simulink model "xblock_half_band_Model"  (Simulink 7.4)
settings: Solver=ode45  StartTime=0.0  StopTime=10.0  RelTol=1e-3
libraries: xbsIndex_r4 x629, casper_library_misc x12
(part 3 of 6)

== system xblock_half_band_Model/Subsystem/parallel_fir/f1/imag_sum ==
  sync : Inport
  din_1 : Inport  Port=2
  din_2 : Inport  Port=3
  din_3 : Inport  Port=4
  din_4 : Inport  Port=5
  din_5 : Inport  Port=6
  din_6 : Inport  Port=7
  din_7 : Inport  Port=8
  din_8 : Inport  Port=9
  din_9 : Inport  Port=10
  sync_delay : xbsIndex_r4/Delay  en=off  latency=4  dbl_ovrd=off  reg_retiming=off  block_type=delay
      settings: block_version=11.4
  zero_in : xbsIndex_r4/Constant  arith_type=Unsigned  const=0  n_bits=18  bin_pt=17  explicit_period=off  period=1  equ=P=C  opselect=C  inp2=PCIN>>17  opr=+  inp1=P  carry=CIN  dbl_ovrd=off  block_type=constant
      settings: block_version=11.4
  sync_out : Outport
  dout : Outport  Port=2
  wires:
  sync/1 -> sync_delay/1
  sync_delay/1 -> sync_out/1

== system xblock_half_band_Model/Subsystem/parallel_fir/f1/real_sum ==
  sync : Inport
  din_1 : Inport  Port=2
  din_2 : Inport  Port=3
  din_3 : Inport  Port=4
  din_4 : Inport  Port=5
  din_5 : Inport  Port=6
  din_6 : Inport  Port=7
  din_7 : Inport  Port=8
  din_8 : Inport  Port=9
  din_9 : Inport  Port=10
  sync_delay : xbsIndex_r4/Delay  en=off  latency=4  dbl_ovrd=off  reg_retiming=off  block_type=delay
      settings: block_version=11.4
  zero_in : xbsIndex_r4/Constant  arith_type=Unsigned  const=0  n_bits=18  bin_pt=17  explicit_period=off  period=1  equ=P=C  opselect=C  inp2=PCIN>>17  opr=+  inp1=P  carry=CIN  dbl_ovrd=off  block_type=constant
      settings: block_version=11.4
  sync_out : Outport
  dout : Outport  Port=2
  wires:
  sync/1 -> sync_delay/1
  sync_delay/1 -> sync_out/1

== system xblock_half_band_Model/Subsystem/parallel_fir1/f0/fir_col1 ==
  real1 : Inport
  imag1 : Inport  Port=2
  fir_tap1 : Subsystem
  real_out1 : Outport
  imag_out1 : Outport  Port=2
  real_sum : Outport  Port=3
  imag_sum : Outport  Port=4
  wires:
  fir_tap1/4(imag) -> imag_sum/1  "xlsub5_fir_tap1_image"
  fir_tap1/1(a_out) -> real_out1/1
  real1/1 -> fir_tap1/1(a)
  imag1/1 -> fir_tap1/2(b)
  fir_tap1/2(b_out) -> imag_out1/1
  fir_tap1/3(real) -> real_sum/1  "xlsub5_fir_tap1_real"

== system xblock_half_band_Model/Subsystem/parallel_fir1/f0/fir_col2 ==
  real1 : Inport
  imag1 : Inport  Port=2
  fir_tap1 : Subsystem
  real_out1 : Outport
  imag_out1 : Outport  Port=2
  real_sum : Outport  Port=3
  imag_sum : Outport  Port=4
  wires:
  fir_tap1/4(imag) -> imag_sum/1  "xlsub5_fir_tap1_image"
  fir_tap1/1(a_out) -> real_out1/1
  real1/1 -> fir_tap1/1(a)
  imag1/1 -> fir_tap1/2(b)
  fir_tap1/2(b_out) -> imag_out1/1
  fir_tap1/3(real) -> real_sum/1  "xlsub5_fir_tap1_real"

== system xblock_half_band_Model/Subsystem/parallel_fir1/f0/fir_col3 ==
  real1 : Inport
  imag1 : Inport  Port=2
  fir_tap1 : Subsystem
  real_out1 : Outport
  imag_out1 : Outport  Port=2
  real_sum : Outport  Port=3
  imag_sum : Outport  Port=4
  wires:
  fir_tap1/4(imag) -> imag_sum/1  "xlsub5_fir_tap1_image"
  fir_tap1/1(a_out) -> real_out1/1
  real1/1 -> fir_tap1/1(a)
  imag1/1 -> fir_tap1/2(b)
  fir_tap1/2(b_out) -> imag_out1/1
  fir_tap1/3(real) -> real_sum/1  "xlsub5_fir_tap1_real"

== system xblock_half_band_Model/Subsystem/parallel_fir1/f0/fir_col4 ==
  real1 : Inport
  imag1 : Inport  Port=2
  fir_tap1 : Subsystem
  real_out1 : Outport
  imag_out1 : Outport  Port=2
  real_sum : Outport  Port=3
  imag_sum : Outport  Port=4
  wires:
  fir_tap1/4(imag) -> imag_sum/1  "xlsub5_fir_tap1_image"
  fir_tap1/1(a_out) -> real_out1/1
  real1/1 -> fir_tap1/1(a)
  imag1/1 -> fir_tap1/2(b)
  fir_tap1/2(b_out) -> imag_out1/1
  fir_tap1/3(real) -> real_sum/1  "xlsub5_fir_tap1_real"

== system xblock_half_band_Model/Subsystem/parallel_fir1/f0/fir_col5 ==
  real1 : Inport
  imag1 : Inport  Port=2
  fir_tap1 : Subsystem
  real_out1 : Outport
  imag_out1 : Outport  Port=2
  real_sum : Outport  Port=3
  imag_sum : Outport  Port=4
  wires:
  fir_tap1/4(imag) -> imag_sum/1  "xlsub5_fir_tap1_image"
  fir_tap1/1(a_out) -> real_out1/1
  real1/1 -> fir_tap1/1(a)
  imag1/1 -> fir_tap1/2(b)
  fir_tap1/2(b_out) -> imag_out1/1
  fir_tap1/3(real) -> real_sum/1  "xlsub5_fir_tap1_real"

== system xblock_half_band_Model/Subsystem/parallel_fir1/f0/fir_col6 ==
  real1 : Inport
  imag1 : Inport  Port=2
  fir_tap1 : Subsystem
  real_out1 : Outport
  imag_out1 : Outport  Port=2
  real_sum : Outport  Port=3
  imag_sum : Outport  Port=4
  wires:
  fir_tap1/4(imag) -> imag_sum/1  "xlsub5_fir_tap1_image"
  fir_tap1/1(a_out) -> real_out1/1
  real1/1 -> fir_tap1/1(a)
  imag1/1 -> fir_tap1/2(b)
  fir_tap1/2(b_out) -> imag_out1/1
  fir_tap1/3(real) -> real_sum/1  "xlsub5_fir_tap1_real"

== system xblock_half_band_Model/Subsystem/parallel_fir1/f0/fir_col7 ==
  real1 : Inport
  imag1 : Inport  Port=2
  fir_tap1 : Subsystem
  real_out1 : Outport
  imag_out1 : Outport  Port=2
  real_sum : Outport  Port=3
  imag_sum : Outport  Port=4
  wires:
  fir_tap1/4(imag) -> imag_sum/1  "xlsub5_fir_tap1_image"
  fir_tap1/1(a_out) -> real_out1/1
  real1/1 -> fir_tap1/1(a)
  imag1/1 -> fir_tap1/2(b)
  fir_tap1/2(b_out) -> imag_out1/1
  fir_tap1/3(real) -> real_sum/1  "xlsub5_fir_tap1_real"

== system xblock_half_band_Model/Subsystem/parallel_fir1/f0/fir_col8 ==
  real1 : Inport
  imag1 : Inport  Port=2
  fir_tap1 : Subsystem
  real_out1 : Outport
  imag_out1 : Outport  Port=2
  real_sum : Outport  Port=3
  imag_sum : Outport  Port=4
  wires:
  fir_tap1/4(imag) -> imag_sum/1  "xlsub5_fir_tap1_image"
  fir_tap1/1(a_out) -> real_out1/1
  real1/1 -> fir_tap1/1(a)
  imag1/1 -> fir_tap1/2(b)
  fir_tap1/2(b_out) -> imag_out1/1
  fir_tap1/3(real) -> real_sum/1  "xlsub5_fir_tap1_real"

== system xblock_half_band_Model/Subsystem/parallel_fir1/f0/imag_sum ==
  sync : Inport
  din_1 : Inport  Port=2
  din_2 : Inport  Port=3
  din_3 : Inport  Port=4
  din_4 : Inport  Port=5
  din_5 : Inport  Port=6
  din_6 : Inport  Port=7
  din_7 : Inport  Port=8
  din_8 : Inport  Port=9
  din_9 : Inport  Port=10
  sync_delay : xbsIndex_r4/Delay  en=off  latency=4  dbl_ovrd=off  reg_retiming=off  block_type=delay
      settings: block_version=11.4
  zero_in : xbsIndex_r4/Constant  arith_type=Unsigned  const=0  n_bits=18  bin_pt=17  explicit_period=off  period=1  equ=P=C  opselect=C  inp2=PCIN>>17  opr=+  inp1=P  carry=CIN  dbl_ovrd=off  block_type=constant
      settings: block_version=11.4
  sync_out : Outport
  dout : Outport  Port=2
  wires:
  sync/1 -> sync_delay/1
  sync_delay/1 -> sync_out/1

== system xblock_half_band_Model/Subsystem/parallel_fir1/f0/real_sum ==
  sync : Inport
  din_1 : Inport  Port=2
  din_2 : Inport  Port=3
  din_3 : Inport  Port=4
  din_4 : Inport  Port=5
  din_5 : Inport  Port=6
  din_6 : Inport  Port=7
  din_7 : Inport  Port=8
  din_8 : Inport  Port=9
  din_9 : Inport  Port=10
  sync_delay : xbsIndex_r4/Delay  en=off  latency=4  dbl_ovrd=off  reg_retiming=off  block_type=delay
      settings: block_version=11.4
  zero_in : xbsIndex_r4/Constant  arith_type=Unsigned  const=0  n_bits=18  bin_pt=17  explicit_period=off  period=1  equ=P=C  opselect=C  inp2=PCIN>>17  opr=+  inp1=P  carry=CIN  dbl_ovrd=off  block_type=constant
      settings: block_version=11.4
  sync_out : Outport
  dout : Outport  Port=2
  wires:
  sync/1 -> sync_delay/1
  sync_delay/1 -> sync_out/1

== system xblock_half_band_Model/Subsystem/parallel_fir1/f0pf1/fir_col1 ==
  real1 : Inport
  imag1 : Inport  Port=2
  fir_tap1 : Subsystem
  real_out1 : Outport
  imag_out1 : Outport  Port=2
  real_sum : Outport  Port=3
  imag_sum : Outport  Port=4
  wires:
  fir_tap1/4(imag) -> imag_sum/1  "xlsub5_fir_tap1_image"
  fir_tap1/1(a_out) -> real_out1/1
  real1/1 -> fir_tap1/1(a)
  imag1/1 -> fir_tap1/2(b)
  fir_tap1/2(b_out) -> imag_out1/1
  fir_tap1/3(real) -> real_sum/1  "xlsub5_fir_tap1_real"

== system xblock_half_band_Model/Subsystem/parallel_fir1/f0pf1/fir_col2 ==
  real1 : Inport
  imag1 : Inport  Port=2
  fir_tap1 : Subsystem
  real_out1 : Outport
  imag_out1 : Outport  Port=2
  real_sum : Outport  Port=3
  imag_sum : Outport  Port=4
  wires:
  fir_tap1/4(imag) -> imag_sum/1  "xlsub5_fir_tap1_image"
  fir_tap1/1(a_out) -> real_out1/1
  real1/1 -> fir_tap1/1(a)
  imag1/1 -> fir_tap1/2(b)
  fir_tap1/2(b_out) -> imag_out1/1
  fir_tap1/3(real) -> real_sum/1  "xlsub5_fir_tap1_real"

== system xblock_half_band_Model/Subsystem/parallel_fir1/f0pf1/fir_col3 ==
  real1 : Inport
  imag1 : Inport  Port=2
  fir_tap1 : Subsystem
  real_out1 : Outport
  imag_out1 : Outport  Port=2
  real_sum : Outport  Port=3
  imag_sum : Outport  Port=4
  wires:
  fir_tap1/4(imag) -> imag_sum/1  "xlsub5_fir_tap1_image"
  fir_tap1/1(a_out) -> real_out1/1
  real1/1 -> fir_tap1/1(a)
  imag1/1 -> fir_tap1/2(b)
  fir_tap1/2(b_out) -> imag_out1/1
  fir_tap1/3(real) -> real_sum/1  "xlsub5_fir_tap1_real"

== system xblock_half_band_Model/Subsystem/parallel_fir1/f0pf1/fir_col4 ==
  real1 : Inport
  imag1 : Inport  Port=2
  fir_tap1 : Subsystem
  real_out1 : Outport
  imag_out1 : Outport  Port=2
  real_sum : Outport  Port=3
  imag_sum : Outport  Port=4
  wires:
  fir_tap1/4(imag) -> imag_sum/1  "xlsub5_fir_tap1_image"
  fir_tap1/1(a_out) -> real_out1/1
  real1/1 -> fir_tap1/1(a)
  imag1/1 -> fir_tap1/2(b)
  fir_tap1/2(b_out) -> imag_out1/1
  fir_tap1/3(real) -> real_sum/1  "xlsub5_fir_tap1_real"

== system xblock_half_band_Model/Subsystem/parallel_fir1/f0pf1/fir_col5 ==
  real1 : Inport
  imag1 : Inport  Port=2
  fir_tap1 : Subsystem
  real_out1 : Outport
  imag_out1 : Outport  Port=2
  real_sum : Outport  Port=3
  imag_sum : Outport  Port=4
  wires:
  fir_tap1/4(imag) -> imag_sum/1  "xlsub5_fir_tap1_image"
  fir_tap1/1(a_out) -> real_out1/1
  real1/1 -> fir_tap1/1(a)
  imag1/1 -> fir_tap1/2(b)
  fir_tap1/2(b_out) -> imag_out1/1
  fir_tap1/3(real) -> real_sum/1  "xlsub5_fir_tap1_real"

== system xblock_half_band_Model/Subsystem/parallel_fir1/f0pf1/imag_sum ==
  sync : Inport
  din_1 : Inport  Port=2
  din_2 : Inport  Port=3
  din_3 : Inport  Port=4
  din_4 : Inport  Port=5
  din_5 : Inport  Port=6
  din_6 : Inport  Port=7
  sync_delay : xbsIndex_r4/Delay  en=off  latency=3  dbl_ovrd=off  reg_retiming=off  block_type=delay
      settings: block_version=11.4
  zero_in : xbsIndex_r4/Constant  arith_type=Unsigned  const=0  n_bits=18  bin_pt=17  explicit_period=off  period=1  equ=P=C  opselect=C  inp2=PCIN>>17  opr=+  inp1=P  carry=CIN  dbl_ovrd=off  block_type=constant
      settings: block_version=11.4
  sync_out : Outport
  dout : Outport  Port=2
  wires:
  sync/1 -> sync_delay/1
  sync_delay/1 -> sync_out/1

== system xblock_half_band_Model/Subsystem/parallel_fir1/f0pf1/real_sum ==
  sync : Inport
  din_1 : Inport  Port=2
  din_2 : Inport  Port=3
  din_3 : Inport  Port=4
  din_4 : Inport  Port=5
  din_5 : Inport  Port=6
  din_6 : Inport  Port=7
  sync_delay : xbsIndex_r4/Delay  en=off  latency=3  dbl_ovrd=off  reg_retiming=off  block_type=delay
      settings: block_version=11.4
  zero_in : xbsIndex_r4/Constant  arith_type=Unsigned  const=0  n_bits=18  bin_pt=17  explicit_period=off  period=1  equ=P=C  opselect=C  inp2=PCIN>>17  opr=+  inp1=P  carry=CIN  dbl_ovrd=off  block_type=constant
      settings: block_version=11.4
  sync_out : Outport
  dout : Outport  Port=2
  wires:
  sync/1 -> sync_delay/1
  sync_delay/1 -> sync_out/1

== system xblock_half_band_Model/Subsystem/parallel_fir1/f1/fir_col1 ==
  real1 : Inport
  imag1 : Inport  Port=2
  fir_tap1 : Subsystem
  real_out1 : Outport
  imag_out1 : Outport  Port=2
  real_sum : Outport  Port=3
  imag_sum : Outport  Port=4
  wires:
  fir_tap1/4(imag) -> imag_sum/1  "xlsub5_fir_tap1_image"
  fir_tap1/1(a_out) -> real_out1/1
  real1/1 -> fir_tap1/1(a)
  imag1/1 -> fir_tap1/2(b)
  fir_tap1/2(b_out) -> imag_out1/1
  fir_tap1/3(real) -> real_sum/1  "xlsub5_fir_tap1_real"

== system xblock_half_band_Model/Subsystem/parallel_fir1/f1/fir_col2 ==
  real1 : Inport
  imag1 : Inport  Port=2
  fir_tap1 : Subsystem
  real_out1 : Outport
  imag_out1 : Outport  Port=2
  real_sum : Outport  Port=3
  imag_sum : Outport  Port=4
  wires:
  fir_tap1/4(imag) -> imag_sum/1  "xlsub5_fir_tap1_image"
  fir_tap1/1(a_out) -> real_out1/1
  real1/1 -> fir_tap1/1(a)
  imag1/1 -> fir_tap1/2(b)
  fir_tap1/2(b_out) -> imag_out1/1
  fir_tap1/3(real) -> real_sum/1  "xlsub5_fir_tap1_real"

== system xblock_half_band_Model/Subsystem/parallel_fir1/f1/fir_col3 ==
  real1 : Inport
  imag1 : Inport  Port=2
  fir_tap1 : Subsystem
  real_out1 : Outport
  imag_out1 : Outport  Port=2
  real_sum : Outport  Port=3
  imag_sum : Outport  Port=4
  wires:
  fir_tap1/4(imag) -> imag_sum/1  "xlsub5_fir_tap1_image"
  fir_tap1/1(a_out) -> real_out1/1
  real1/1 -> fir_tap1/1(a)
  imag1/1 -> fir_tap1/2(b)
  fir_tap1/2(b_out) -> imag_out1/1
  fir_tap1/3(real) -> real_sum/1  "xlsub5_fir_tap1_real"

== system xblock_half_band_Model/Subsystem/parallel_fir1/f1/fir_col4 ==
  real1 : Inport
  imag1 : Inport  Port=2
  fir_tap1 : Subsystem
  real_out1 : Outport
  imag_out1 : Outport  Port=2
  real_sum : Outport  Port=3
  imag_sum : Outport  Port=4
  wires:
  fir_tap1/4(imag) -> imag_sum/1  "xlsub5_fir_tap1_image"
  fir_tap1/1(a_out) -> real_out1/1
  real1/1 -> fir_tap1/1(a)
  imag1/1 -> fir_tap1/2(b)
  fir_tap1/2(b_out) -> imag_out1/1
  fir_tap1/3(real) -> real_sum/1  "xlsub5_fir_tap1_real"

== system xblock_half_band_Model/Subsystem/parallel_fir1/f1/fir_col5 ==
  real1 : Inport
  imag1 : Inport  Port=2
  fir_tap1 : Subsystem
  real_out1 : Outport
  imag_out1 : Outport  Port=2
  real_sum : Outport  Port=3
  imag_sum : Outport  Port=4
  wires:
  fir_tap1/4(imag) -> imag_sum/1  "xlsub5_fir_tap1_image"
  fir_tap1/1(a_out) -> real_out1/1
  real1/1 -> fir_tap1/1(a)
  imag1/1 -> fir_tap1/2(b)
  fir_tap1/2(b_out) -> imag_out1/1
  fir_tap1/3(real) -> real_sum/1  "xlsub5_fir_tap1_real"

== system xblock_half_band_Model/Subsystem/parallel_fir1/f1/fir_col6 ==
  real1 : Inport
  imag1 : Inport  Port=2
  fir_tap1 : Subsystem
  real_out1 : Outport
  imag_out1 : Outport  Port=2
  real_sum : Outport  Port=3
  imag_sum : Outport  Port=4
  wires:
  fir_tap1/4(imag) -> imag_sum/1  "xlsub5_fir_tap1_image"
  fir_tap1/1(a_out) -> real_out1/1
  real1/1 -> fir_tap1/1(a)
  imag1/1 -> fir_tap1/2(b)
  fir_tap1/2(b_out) -> imag_out1/1
  fir_tap1/3(real) -> real_sum/1  "xlsub5_fir_tap1_real"

== system xblock_half_band_Model/Subsystem/parallel_fir1/f1/fir_col7 ==
  real1 : Inport
  imag1 : Inport  Port=2
  fir_tap1 : Subsystem
  real_out1 : Outport
  imag_out1 : Outport  Port=2
  real_sum : Outport  Port=3
  imag_sum : Outport  Port=4
  wires:
  fir_tap1/4(imag) -> imag_sum/1  "xlsub5_fir_tap1_image"
  fir_tap1/1(a_out) -> real_out1/1
  real1/1 -> fir_tap1/1(a)
  imag1/1 -> fir_tap1/2(b)
  fir_tap1/2(b_out) -> imag_out1/1
  fir_tap1/3(real) -> real_sum/1  "xlsub5_fir_tap1_real"

== system xblock_half_band_Model/Subsystem/parallel_fir1/f1/fir_col8 ==
  real1 : Inport
  imag1 : Inport  Port=2
  fir_tap1 : Subsystem
  real_out1 : Outport
  imag_out1 : Outport  Port=2
  real_sum : Outport  Port=3
  imag_sum : Outport  Port=4
  wires:
  fir_tap1/4(imag) -> imag_sum/1  "xlsub5_fir_tap1_image"
  fir_tap1/1(a_out) -> real_out1/1
  real1/1 -> fir_tap1/1(a)
  imag1/1 -> fir_tap1/2(b)
  fir_tap1/2(b_out) -> imag_out1/1
  fir_tap1/3(real) -> real_sum/1  "xlsub5_fir_tap1_real"

== system xblock_half_band_Model/Subsystem/parallel_fir1/f1/imag_sum ==
  sync : Inport
  din_1 : Inport  Port=2
  din_2 : Inport  Port=3
  din_3 : Inport  Port=4
  din_4 : Inport  Port=5
  din_5 : Inport  Port=6
  din_6 : Inport  Port=7
  din_7 : Inport  Port=8
  din_8 : Inport  Port=9
  din_9 : Inport  Port=10
  sync_delay : xbsIndex_r4/Delay  en=off  latency=4  dbl_ovrd=off  reg_retiming=off  block_type=delay
      settings: block_version=11.4
  zero_in : xbsIndex_r4/Constant  arith_type=Unsigned  const=0  n_bits=18  bin_pt=17  explicit_period=off  period=1  equ=P=C  opselect=C  inp2=PCIN>>17  opr=+  inp1=P  carry=CIN  dbl_ovrd=off  block_type=constant
      settings: block_version=11.4
  sync_out : Outport
  dout : Outport  Port=2
  wires:
  sync/1 -> sync_delay/1
  sync_delay/1 -> sync_out/1

== system xblock_half_band_Model/Subsystem/parallel_fir1/f1/real_sum ==
  sync : Inport
  din_1 : Inport  Port=2
  din_2 : Inport  Port=3
  din_3 : Inport  Port=4
  din_4 : Inport  Port=5
  din_5 : Inport  Port=6
  din_6 : Inport  Port=7
  din_7 : Inport  Port=8
  din_8 : Inport  Port=9
  din_9 : Inport  Port=10
  sync_delay : xbsIndex_r4/Delay  en=off  latency=4  dbl_ovrd=off  reg_retiming=off  block_type=delay
      settings: block_version=11.4
  zero_in : xbsIndex_r4/Constant  arith_type=Unsigned  const=0  n_bits=18  bin_pt=17  explicit_period=off  period=1  equ=P=C  opselect=C  inp2=PCIN>>17  opr=+  inp1=P  carry=CIN  dbl_ovrd=off  block_type=constant
      settings: block_version=11.4
  sync_out : Outport
  dout : Outport  Port=2
  wires:
  sync/1 -> sync_delay/1
  sync_delay/1 -> sync_out/1

== system xblock_half_band_Model/Subsystem/parallel_fir2/f0/fir_col1 ==
  real1 : Inport
  imag1 : Inport  Port=2
  fir_tap1 : Subsystem
  real_out1 : Outport
  imag_out1 : Outport  Port=2
  real_sum : Outport  Port=3
  imag_sum : Outport  Port=4
  wires:
  fir_tap1/4(imag) -> imag_sum/1  "xlsub5_fir_tap1_image"
  fir_tap1/1(a_out) -> real_out1/1
  real1/1 -> fir_tap1/1(a)
  imag1/1 -> fir_tap1/2(b)
  fir_tap1/2(b_out) -> imag_out1/1
  fir_tap1/3(real) -> real_sum/1  "xlsub5_fir_tap1_real"

== system xblock_half_band_Model/Subsystem/parallel_fir2/f0/fir_col2 ==
  real1 : Inport
  imag1 : Inport  Port=2
  fir_tap1 : Subsystem
  real_out1 : Outport
  imag_out1 : Outport  Port=2
  real_sum : Outport  Port=3
  imag_sum : Outport  Port=4
  wires:
  fir_tap1/4(imag) -> imag_sum/1  "xlsub5_fir_tap1_image"
  fir_tap1/1(a_out) -> real_out1/1
  real1/1 -> fir_tap1/1(a)
  imag1/1 -> fir_tap1/2(b)
  fir_tap1/2(b_out) -> imag_out1/1
  fir_tap1/3(real) -> real_sum/1  "xlsub5_fir_tap1_real"

== system xblock_half_band_Model/Subsystem/parallel_fir2/f0/fir_col3 ==
  real1 : Inport
  imag1 : Inport  Port=2
  fir_tap1 : Subsystem
  real_out1 : Outport
  imag_out1 : Outport  Port=2
  real_sum : Outport  Port=3
  imag_sum : Outport  Port=4
  wires:
  fir_tap1/4(imag) -> imag_sum/1  "xlsub5_fir_tap1_image"
  fir_tap1/1(a_out) -> real_out1/1
  real1/1 -> fir_tap1/1(a)
  imag1/1 -> fir_tap1/2(b)
  fir_tap1/2(b_out) -> imag_out1/1
  fir_tap1/3(real) -> real_sum/1  "xlsub5_fir_tap1_real"

== system xblock_half_band_Model/Subsystem/parallel_fir2/f0/fir_col4 ==
  real1 : Inport
  imag1 : Inport  Port=2
  fir_tap1 : Subsystem
  real_out1 : Outport
  imag_out1 : Outport  Port=2
  real_sum : Outport  Port=3
  imag_sum : Outport  Port=4
  wires:
  fir_tap1/4(imag) -> imag_sum/1  "xlsub5_fir_tap1_image"
  fir_tap1/1(a_out) -> real_out1/1
  real1/1 -> fir_tap1/1(a)
  imag1/1 -> fir_tap1/2(b)
  fir_tap1/2(b_out) -> imag_out1/1
  fir_tap1/3(real) -> real_sum/1  "xlsub5_fir_tap1_real"

== system xblock_half_band_Model/Subsystem/parallel_fir2/f0/fir_col5 ==
  real1 : Inport
  imag1 : Inport  Port=2
  fir_tap1 : Subsystem
  real_out1 : Outport
  imag_out1 : Outport  Port=2
  real_sum : Outport  Port=3
  imag_sum : Outport  Port=4
  wires:
  fir_tap1/4(imag) -> imag_sum/1  "xlsub5_fir_tap1_image"
  fir_tap1/1(a_out) -> real_out1/1
  real1/1 -> fir_tap1/1(a)
  imag1/1 -> fir_tap1/2(b)
  fir_tap1/2(b_out) -> imag_out1/1
  fir_tap1/3(real) -> real_sum/1  "xlsub5_fir_tap1_real"

== system xblock_half_band_Model/Subsystem/parallel_fir2/f0/fir_col6 ==
  real1 : Inport
  imag1 : Inport  Port=2
  fir_tap1 : Subsystem
  real_out1 : Outport
  imag_out1 : Outport  Port=2
  real_sum : Outport  Port=3
  imag_sum : Outport  Port=4
  wires:
  fir_tap1/4(imag) -> imag_sum/1  "xlsub5_fir_tap1_image"
  fir_tap1/1(a_out) -> real_out1/1
  real1/1 -> fir_tap1/1(a)
  imag1/1 -> fir_tap1/2(b)
  fir_tap1/2(b_out) -> imag_out1/1
  fir_tap1/3(real) -> real_sum/1  "xlsub5_fir_tap1_real"

== system xblock_half_band_Model/Subsystem/parallel_fir2/f0/fir_col7 ==
  real1 : Inport
  imag1 : Inport  Port=2
  fir_tap1 : Subsystem
  real_out1 : Outport
  imag_out1 : Outport  Port=2
  real_sum : Outport  Port=3
  imag_sum : Outport  Port=4
  wires:
  fir_tap1/4(imag) -> imag_sum/1  "xlsub5_fir_tap1_image"
  fir_tap1/1(a_out) -> real_out1/1
  real1/1 -> fir_tap1/1(a)
  imag1/1 -> fir_tap1/2(b)
  fir_tap1/2(b_out) -> imag_out1/1
  fir_tap1/3(real) -> real_sum/1  "xlsub5_fir_tap1_real"

== system xblock_half_band_Model/Subsystem/parallel_fir2/f0/fir_col8 ==
  real1 : Inport
  imag1 : Inport  Port=2
  fir_tap1 : Subsystem
  real_out1 : Outport
  imag_out1 : Outport  Port=2
  real_sum : Outport  Port=3
  imag_sum : Outport  Port=4
  wires:
  fir_tap1/4(imag) -> imag_sum/1  "xlsub5_fir_tap1_image"
  fir_tap1/1(a_out) -> real_out1/1
  real1/1 -> fir_tap1/1(a)
  imag1/1 -> fir_tap1/2(b)
  fir_tap1/2(b_out) -> imag_out1/1
  fir_tap1/3(real) -> real_sum/1  "xlsub5_fir_tap1_real"

== system xblock_half_band_Model/Subsystem/parallel_fir2/f0/imag_sum ==
  sync : Inport
  din_1 : Inport  Port=2
  din_2 : Inport  Port=3
  din_3 : Inport  Port=4
  din_4 : Inport  Port=5
  din_5 : Inport  Port=6
  din_6 : Inport  Port=7
  din_7 : Inport  Port=8
  din_8 : Inport  Port=9
  din_9 : Inport  Port=10
  sync_delay : xbsIndex_r4/Delay  en=off  latency=4  dbl_ovrd=off  reg_retiming=off  block_type=delay
      settings: block_version=11.4
  zero_in : xbsIndex_r4/Constant  arith_type=Unsigned  const=0  n_bits=18  bin_pt=17  explicit_period=off  period=1  equ=P=C  opselect=C  inp2=PCIN>>17  opr=+  inp1=P  carry=CIN  dbl_ovrd=off  block_type=constant
      settings: block_version=11.4
  sync_out : Outport
  dout : Outport  Port=2
  wires:
  sync/1 -> sync_delay/1
  sync_delay/1 -> sync_out/1

== system xblock_half_band_Model/Subsystem/parallel_fir2/f0/real_sum ==
  sync : Inport
  din_1 : Inport  Port=2
  din_2 : Inport  Port=3
  din_3 : Inport  Port=4
  din_4 : Inport  Port=5
  din_5 : Inport  Port=6
  din_6 : Inport  Port=7
  din_7 : Inport  Port=8
  din_8 : Inport  Port=9
  din_9 : Inport  Port=10
  sync_delay : xbsIndex_r4/Delay  en=off  latency=4  dbl_ovrd=off  reg_retiming=off  block_type=delay
      settings: block_version=11.4
  zero_in : xbsIndex_r4/Constant  arith_type=Unsigned  const=0  n_bits=18  bin_pt=17  explicit_period=off  period=1  equ=P=C  opselect=C  inp2=PCIN>>17  opr=+  inp1=P  carry=CIN  dbl_ovrd=off  block_type=constant
      settings: block_version=11.4
  sync_out : Outport
  dout : Outport  Port=2
  wires:
  sync/1 -> sync_delay/1
  sync_delay/1 -> sync_out/1

== system xblock_half_band_Model/Subsystem/parallel_fir2/f0pf1/fir_col1 ==
  real1 : Inport
  imag1 : Inport  Port=2
  fir_tap1 : Subsystem
  real_out1 : Outport
  imag_out1 : Outport  Port=2
  real_sum : Outport  Port=3
  imag_sum : Outport  Port=4
  wires:
  fir_tap1/4(imag) -> imag_sum/1  "xlsub5_fir_tap1_image"
  fir_tap1/1(a_out) -> real_out1/1
  real1/1 -> fir_tap1/1(a)
  imag1/1 -> fir_tap1/2(b)
  fir_tap1/2(b_out) -> imag_out1/1
  fir_tap1/3(real) -> real_sum/1  "xlsub5_fir_tap1_real"

== system xblock_half_band_Model/Subsystem/parallel_fir2/f0pf1/fir_col2 ==
  real1 : Inport
  imag1 : Inport  Port=2
  fir_tap1 : Subsystem
  real_out1 : Outport
  imag_out1 : Outport  Port=2
  real_sum : Outport  Port=3
  imag_sum : Outport  Port=4
  wires:
  fir_tap1/4(imag) -> imag_sum/1  "xlsub5_fir_tap1_image"
  fir_tap1/1(a_out) -> real_out1/1
  real1/1 -> fir_tap1/1(a)
  imag1/1 -> fir_tap1/2(b)
  fir_tap1/2(b_out) -> imag_out1/1
  fir_tap1/3(real) -> real_sum/1  "xlsub5_fir_tap1_real"

== system xblock_half_band_Model/Subsystem/parallel_fir2/f0pf1/fir_col3 ==
  real1 : Inport
  imag1 : Inport  Port=2
  fir_tap1 : Subsystem
  real_out1 : Outport
  imag_out1 : Outport  Port=2
  real_sum : Outport  Port=3
  imag_sum : Outport  Port=4
  wires:
  fir_tap1/4(imag) -> imag_sum/1  "xlsub5_fir_tap1_image"
  fir_tap1/1(a_out) -> real_out1/1
  real1/1 -> fir_tap1/1(a)
  imag1/1 -> fir_tap1/2(b)
  fir_tap1/2(b_out) -> imag_out1/1
  fir_tap1/3(real) -> real_sum/1  "xlsub5_fir_tap1_real"

== system xblock_half_band_Model/Subsystem/parallel_fir2/f0pf1/fir_col4 ==
  real1 : Inport
  imag1 : Inport  Port=2
  fir_tap1 : Subsystem
  real_out1 : Outport
  imag_out1 : Outport  Port=2
  real_sum : Outport  Port=3
  imag_sum : Outport  Port=4
  wires:
  fir_tap1/4(imag) -> imag_sum/1  "xlsub5_fir_tap1_image"
  fir_tap1/1(a_out) -> real_out1/1
  real1/1 -> fir_tap1/1(a)
  imag1/1 -> fir_tap1/2(b)
  fir_tap1/2(b_out) -> imag_out1/1
  fir_tap1/3(real) -> real_sum/1  "xlsub5_fir_tap1_real"

== system xblock_half_band_Model/Subsystem/parallel_fir2/f0pf1/fir_col5 ==
  real1 : Inport
  imag1 : Inport  Port=2
  fir_tap1 : Subsystem
  real_out1 : Outport
  imag_out1 : Outport  Port=2
  real_sum : Outport  Port=3
  imag_sum : Outport  Port=4
  wires:
  fir_tap1/4(imag) -> imag_sum/1  "xlsub5_fir_tap1_image"
  fir_tap1/1(a_out) -> real_out1/1
  real1/1 -> fir_tap1/1(a)
  imag1/1 -> fir_tap1/2(b)
  fir_tap1/2(b_out) -> imag_out1/1
  fir_tap1/3(real) -> real_sum/1  "xlsub5_fir_tap1_real"

== system xblock_half_band_Model/Subsystem/parallel_fir2/f0pf1/imag_sum ==
  sync : Inport
  din_1 : Inport  Port=2
  din_2 : Inport  Port=3
  din_3 : Inport  Port=4
  din_4 : Inport  Port=5
  din_5 : Inport  Port=6
  din_6 : Inport  Port=7
  sync_delay : xbsIndex_r4/Delay  en=off  latency=3  dbl_ovrd=off  reg_retiming=off  block_type=delay
      settings: block_version=11.4
  zero_in : xbsIndex_r4/Constant  arith_type=Unsigned  const=0  n_bits=18  bin_pt=17  explicit_period=off  period=1  equ=P=C  opselect=C  inp2=PCIN>>17  opr=+  inp1=P  carry=CIN  dbl_ovrd=off  block_type=constant
      settings: block_version=11.4
  sync_out : Outport
  dout : Outport  Port=2
  wires:
  sync/1 -> sync_delay/1
  sync_delay/1 -> sync_out/1

== system xblock_half_band_Model/Subsystem/parallel_fir2/f0pf1/real_sum ==
  sync : Inport
  din_1 : Inport  Port=2
  din_2 : Inport  Port=3
  din_3 : Inport  Port=4
  din_4 : Inport  Port=5
  din_5 : Inport  Port=6
  din_6 : Inport  Port=7
  sync_delay : xbsIndex_r4/Delay  en=off  latency=3  dbl_ovrd=off  reg_retiming=off  block_type=delay
      settings: block_version=11.4
  zero_in : xbsIndex_r4/Constant  arith_type=Unsigned  const=0  n_bits=18  bin_pt=17  explicit_period=off  period=1  equ=P=C  opselect=C  inp2=PCIN>>17  opr=+  inp1=P  carry=CIN  dbl_ovrd=off  block_type=constant
      settings: block_version=11.4
  sync_out : Outport
  dout : Outport  Port=2
  wires:
  sync/1 -> sync_delay/1
  sync_delay/1 -> sync_out/1

== system xblock_half_band_Model/Subsystem/parallel_fir2/f1/fir_col1 ==
  real1 : Inport
  imag1 : Inport  Port=2
  fir_tap1 : Subsystem
  real_out1 : Outport
  imag_out1 : Outport  Port=2
  real_sum : Outport  Port=3
  imag_sum : Outport  Port=4
  wires:
  fir_tap1/4(imag) -> imag_sum/1  "xlsub5_fir_tap1_image"
  fir_tap1/1(a_out) -> real_out1/1
  real1/1 -> fir_tap1/1(a)
  imag1/1 -> fir_tap1/2(b)
  fir_tap1/2(b_out) -> imag_out1/1
  fir_tap1/3(real) -> real_sum/1  "xlsub5_fir_tap1_real"

== system xblock_half_band_Model/Subsystem/parallel_fir2/f1/fir_col2 ==
  real1 : Inport
  imag1 : Inport  Port=2
  fir_tap1 : Subsystem
  real_out1 : Outport
  imag_out1 : Outport  Port=2
  real_sum : Outport  Port=3
  imag_sum : Outport  Port=4
  wires:
  fir_tap1/4(imag) -> imag_sum/1  "xlsub5_fir_tap1_image"
  fir_tap1/1(a_out) -> real_out1/1
  real1/1 -> fir_tap1/1(a)
  imag1/1 -> fir_tap1/2(b)
  fir_tap1/2(b_out) -> imag_out1/1
  fir_tap1/3(real) -> real_sum/1  "xlsub5_fir_tap1_real"

== system xblock_half_band_Model/Subsystem/parallel_fir2/f1/fir_col3 ==
  real1 : Inport
  imag1 : Inport  Port=2
  fir_tap1 : Subsystem
  real_out1 : Outport
  imag_out1 : Outport  Port=2
  real_sum : Outport  Port=3
  imag_sum : Outport  Port=4
  wires:
  fir_tap1/4(imag) -> imag_sum/1  "xlsub5_fir_tap1_image"
  fir_tap1/1(a_out) -> real_out1/1
  real1/1 -> fir_tap1/1(a)
  imag1/1 -> fir_tap1/2(b)
  fir_tap1/2(b_out) -> imag_out1/1
  fir_tap1/3(real) -> real_sum/1  "xlsub5_fir_tap1_real"

== system xblock_half_band_Model/Subsystem/parallel_fir2/f1/fir_col4 ==
  real1 : Inport
  imag1 : Inport  Port=2
  fir_tap1 : Subsystem
  real_out1 : Outport
  imag_out1 : Outport  Port=2
  real_sum : Outport  Port=3
  imag_sum : Outport  Port=4
  wires:
  fir_tap1/4(imag) -> imag_sum/1  "xlsub5_fir_tap1_image"
  fir_tap1/1(a_out) -> real_out1/1
  real1/1 -> fir_tap1/1(a)
  imag1/1 -> fir_tap1/2(b)
  fir_tap1/2(b_out) -> imag_out1/1
  fir_tap1/3(real) -> real_sum/1  "xlsub5_fir_tap1_real"

== system xblock_half_band_Model/Subsystem/parallel_fir2/f1/fir_col5 ==
  real1 : Inport
  imag1 : Inport  Port=2
  fir_tap1 : Subsystem
  real_out1 : Outport
  imag_out1 : Outport  Port=2
  real_sum : Outport  Port=3
  imag_sum : Outport  Port=4
  wires:
  fir_tap1/4(imag) -> imag_sum/1  "xlsub5_fir_tap1_image"
  fir_tap1/1(a_out) -> real_out1/1
  real1/1 -> fir_tap1/1(a)
  imag1/1 -> fir_tap1/2(b)
  fir_tap1/2(b_out) -> imag_out1/1
  fir_tap1/3(real) -> real_sum/1  "xlsub5_fir_tap1_real"

== system xblock_half_band_Model/Subsystem/parallel_fir2/f1/fir_col6 ==
  real1 : Inport
  imag1 : Inport  Port=2
  fir_tap1 : Subsystem
  real_out1 : Outport
  imag_out1 : Outport  Port=2
  real_sum : Outport  Port=3
  imag_sum : Outport  Port=4
  wires:
  fir_tap1/4(imag) -> imag_sum/1  "xlsub5_fir_tap1_image"
  fir_tap1/1(a_out) -> real_out1/1
  real1/1 -> fir_tap1/1(a)
  imag1/1 -> fir_tap1/2(b)
  fir_tap1/2(b_out) -> imag_out1/1
  fir_tap1/3(real) -> real_sum/1  "xlsub5_fir_tap1_real"

== system xblock_half_band_Model/Subsystem/parallel_fir2/f1/fir_col7 ==
  real1 : Inport
  imag1 : Inport  Port=2
  fir_tap1 : Subsystem
  real_out1 : Outport
  imag_out1 : Outport  Port=2
  real_sum : Outport  Port=3
  imag_sum : Outport  Port=4
  wires:
  fir_tap1/4(imag) -> imag_sum/1  "xlsub5_fir_tap1_image"
  fir_tap1/1(a_out) -> real_out1/1
  real1/1 -> fir_tap1/1(a)
  imag1/1 -> fir_tap1/2(b)
  fir_tap1/2(b_out) -> imag_out1/1
  fir_tap1/3(real) -> real_sum/1  "xlsub5_fir_tap1_real"

== system xblock_half_band_Model/Subsystem/parallel_fir2/f1/fir_col8 ==
  real1 : Inport
  imag1 : Inport  Port=2
  fir_tap1 : Subsystem
  real_out1 : Outport
  imag_out1 : Outport  Port=2
  real_sum : Outport  Port=3
  imag_sum : Outport  Port=4
  wires:
  fir_tap1/4(imag) -> imag_sum/1  "xlsub5_fir_tap1_image"
  fir_tap1/1(a_out) -> real_out1/1
  real1/1 -> fir_tap1/1(a)
  imag1/1 -> fir_tap1/2(b)
  fir_tap1/2(b_out) -> imag_out1/1
  fir_tap1/3(real) -> real_sum/1  "xlsub5_fir_tap1_real"

== system xblock_half_band_Model/Subsystem/parallel_fir2/f1/imag_sum ==
  sync : Inport
  din_1 : Inport  Port=2
  din_2 : Inport  Port=3
  din_3 : Inport  Port=4
  din_4 : Inport  Port=5
  din_5 : Inport  Port=6
  din_6 : Inport  Port=7
  din_7 : Inport  Port=8
  din_8 : Inport  Port=9
  din_9 : Inport  Port=10
  sync_delay : xbsIndex_r4/Delay  en=off  latency=4  dbl_ovrd=off  reg_retiming=off  block_type=delay
      settings: block_version=11.4
  zero_in : xbsIndex_r4/Constant  arith_type=Unsigned  const=0  n_bits=18  bin_pt=17  explicit_period=off  period=1  equ=P=C  opselect=C  inp2=PCIN>>17  opr=+  inp1=P  carry=CIN  dbl_ovrd=off  block_type=constant
      settings: block_version=11.4
  sync_out : Outport
  dout : Outport  Port=2
  wires:
  sync/1 -> sync_delay/1
  sync_delay/1 -> sync_out/1

== system xblock_half_band_Model/Subsystem/parallel_fir2/f1/real_sum ==
  sync : Inport
  din_1 : Inport  Port=2
  din_2 : Inport  Port=3
  din_3 : Inport  Port=4
  din_4 : Inport  Port=5
  din_5 : Inport  Port=6
  din_6 : Inport  Port=7
  din_7 : Inport  Port=8
  din_8 : Inport  Port=9
  din_9 : Inport  Port=10
  sync_delay : xbsIndex_r4/Delay  en=off  latency=4  dbl_ovrd=off  reg_retiming=off  block_type=delay
      settings: block_version=11.4
  zero_in : xbsIndex_r4/Constant  arith_type=Unsigned  const=0  n_bits=18  bin_pt=17  explicit_period=off  period=1  equ=P=C  opselect=C  inp2=PCIN>>17  opr=+  inp1=P  carry=CIN  dbl_ovrd=off  block_type=constant
      settings: block_version=11.4
  sync_out : Outport
  dout : Outport  Port=2
  wires:
  sync/1 -> sync_delay/1
  sync_delay/1 -> sync_out/1

== system xblock_half_band_Model/Subsystem/parallel_fir3/f0/fir_col1 ==
  real1 : Inport
  imag1 : Inport  Port=2
  fir_tap1 : Subsystem
  real_out1 : Outport
  imag_out1 : Outport  Port=2
  real_sum : Outport  Port=3
  imag_sum : Outport  Port=4
  wires:
  fir_tap1/4(imag) -> imag_sum/1  "xlsub5_fir_tap1_image"
  fir_tap1/1(a_out) -> real_out1/1
  real1/1 -> fir_tap1/1(a)
  imag1/1 -> fir_tap1/2(b)
  fir_tap1/2(b_out) -> imag_out1/1
  fir_tap1/3(real) -> real_sum/1  "xlsub5_fir_tap1_real"

== system xblock_half_band_Model/Subsystem/parallel_fir3/f0/fir_col2 ==
  real1 : Inport
  imag1 : Inport  Port=2
  fir_tap1 : Subsystem
  real_out1 : Outport
  imag_out1 : Outport  Port=2
  real_sum : Outport  Port=3
  imag_sum : Outport  Port=4
  wires:
  fir_tap1/4(imag) -> imag_sum/1  "xlsub5_fir_tap1_image"
  fir_tap1/1(a_out) -> real_out1/1
  real1/1 -> fir_tap1/1(a)
  imag1/1 -> fir_tap1/2(b)
  fir_tap1/2(b_out) -> imag_out1/1
  fir_tap1/3(real) -> real_sum/1  "xlsub5_fir_tap1_real"

== system xblock_half_band_Model/Subsystem/parallel_fir3/f0/fir_col3 ==
  real1 : Inport
  imag1 : Inport  Port=2
  fir_tap1 : Subsystem
  real_out1 : Outport
  imag_out1 : Outport  Port=2
  real_sum : Outport  Port=3
  imag_sum : Outport  Port=4
  wires:
  fir_tap1/4(imag) -> imag_sum/1  "xlsub5_fir_tap1_image"
  fir_tap1/1(a_out) -> real_out1/1
  real1/1 -> fir_tap1/1(a)
  imag1/1 -> fir_tap1/2(b)
  fir_tap1/2(b_out) -> imag_out1/1
  fir_tap1/3(real) -> real_sum/1  "xlsub5_fir_tap1_real"

== system xblock_half_band_Model/Subsystem/parallel_fir3/f0/fir_col4 ==
  real1 : Inport
  imag1 : Inport  Port=2
  fir_tap1 : Subsystem
  real_out1 : Outport
  imag_out1 : Outport  Port=2
  real_sum : Outport  Port=3
  imag_sum : Outport  Port=4
  wires:
  fir_tap1/4(imag) -> imag_sum/1  "xlsub5_fir_tap1_image"
  fir_tap1/1(a_out) -> real_out1/1
  real1/1 -> fir_tap1/1(a)
  imag1/1 -> fir_tap1/2(b)
  fir_tap1/2(b_out) -> imag_out1/1
  fir_tap1/3(real) -> real_sum/1  "xlsub5_fir_tap1_real"

== system xblock_half_band_Model/Subsystem/parallel_fir3/f0/fir_col5 ==
  real1 : Inport
  imag1 : Inport  Port=2
  fir_tap1 : Subsystem
  real_out1 : Outport
  imag_out1 : Outport  Port=2
  real_sum : Outport  Port=3
  imag_sum : Outport  Port=4
  wires:
  fir_tap1/4(imag) -> imag_sum/1  "xlsub5_fir_tap1_image"
  fir_tap1/1(a_out) -> real_out1/1
  real1/1 -> fir_tap1/1(a)
  imag1/1 -> fir_tap1/2(b)
  fir_tap1/2(b_out) -> imag_out1/1
  fir_tap1/3(real) -> real_sum/1  "xlsub5_fir_tap1_real"

== system xblock_half_band_Model/Subsystem/parallel_fir3/f0/fir_col6 ==
  real1 : Inport
  imag1 : Inport  Port=2
  fir_tap1 : Subsystem
  real_out1 : Outport
  imag_out1 : Outport  Port=2
  real_sum : Outport  Port=3
  imag_sum : Outport  Port=4
  wires:
  fir_tap1/4(imag) -> imag_sum/1  "xlsub5_fir_tap1_image"
  fir_tap1/1(a_out) -> real_out1/1
  real1/1 -> fir_tap1/1(a)
  imag1/1 -> fir_tap1/2(b)
  fir_tap1/2(b_out) -> imag_out1/1
  fir_tap1/3(real) -> real_sum/1  "xlsub5_fir_tap1_real"

== system xblock_half_band_Model/Subsystem/parallel_fir3/f0/fir_col7 ==
  real1 : Inport
  imag1 : Inport  Port=2
  fir_tap1 : Subsystem
  real_out1 : Outport
  imag_out1 : Outport  Port=2
  real_sum : Outport  Port=3
  imag_sum : Outport  Port=4
  wires:
  fir_tap1/4(imag) -> imag_sum/1  "xlsub5_fir_tap1_image"
  fir_tap1/1(a_out) -> real_out1/1
  real1/1 -> fir_tap1/1(a)
  imag1/1 -> fir_tap1/2(b)
  fir_tap1/2(b_out) -> imag_out1/1
  fir_tap1/3(real) -> real_sum/1  "xlsub5_fir_tap1_real"

== system xblock_half_band_Model/Subsystem/parallel_fir3/f0/fir_col8 ==
  real1 : Inport
  imag1 : Inport  Port=2
  fir_tap1 : Subsystem
  real_out1 : Outport
  imag_out1 : Outport  Port=2
  real_sum : Outport  Port=3
  imag_sum : Outport  Port=4
  wires:
  fir_tap1/4(imag) -> imag_sum/1  "xlsub5_fir_tap1_image"
  fir_tap1/1(a_out) -> real_out1/1
  real1/1 -> fir_tap1/1(a)
  imag1/1 -> fir_tap1/2(b)
  fir_tap1/2(b_out) -> imag_out1/1
  fir_tap1/3(real) -> real_sum/1  "xlsub5_fir_tap1_real"

== system xblock_half_band_Model/Subsystem/parallel_fir3/f0/imag_sum ==
  sync : Inport
  din_1 : Inport  Port=2
  din_2 : Inport  Port=3
  din_3 : Inport  Port=4
  din_4 : Inport  Port=5
  din_5 : Inport  Port=6
  din_6 : Inport  Port=7
  din_7 : Inport  Port=8
  din_8 : Inport  Port=9
  din_9 : Inport  Port=10
  sync_delay : xbsIndex_r4/Delay  en=off  latency=4  dbl_ovrd=off  reg_retiming=off  block_type=delay
      settings: block_version=11.4
  zero_in : xbsIndex_r4/Constant  arith_type=Unsigned  const=0  n_bits=18  bin_pt=17  explicit_period=off  period=1  equ=P=C  opselect=C  inp2=PCIN>>17  opr=+  inp1=P  carry=CIN  dbl_ovrd=off  block_type=constant
      settings: block_version=11.4
  sync_out : Outport
  dout : Outport  Port=2
  wires:
  sync/1 -> sync_delay/1
  sync_delay/1 -> sync_out/1

== system xblock_half_band_Model/Subsystem/parallel_fir3/f0/real_sum ==
  sync : Inport
  din_1 : Inport  Port=2
  din_2 : Inport  Port=3
  din_3 : Inport  Port=4
  din_4 : Inport  Port=5
  din_5 : Inport  Port=6
  din_6 : Inport  Port=7
  din_7 : Inport  Port=8
  din_8 : Inport  Port=9
  din_9 : Inport  Port=10
  sync_delay : xbsIndex_r4/Delay  en=off  latency=4  dbl_ovrd=off  reg_retiming=off  block_type=delay
      settings: block_version=11.4
  zero_in : xbsIndex_r4/Constant  arith_type=Unsigned  const=0  n_bits=18  bin_pt=17  explicit_period=off  period=1  equ=P=C  opselect=C  inp2=PCIN>>17  opr=+  inp1=P  carry=CIN  dbl_ovrd=off  block_type=constant
      settings: block_version=11.4
  sync_out : Outport
  dout : Outport  Port=2
  wires:
  sync/1 -> sync_delay/1
  sync_delay/1 -> sync_out/1

== system xblock_half_band_Model/Subsystem/parallel_fir3/f0pf1/fir_col1 ==
  real1 : Inport
  imag1 : Inport  Port=2
  fir_tap1 : Subsystem
  real_out1 : Outport
  imag_out1 : Outport  Port=2
  real_sum : Outport  Port=3
  imag_sum : Outport  Port=4
  wires:
  fir_tap1/4(imag) -> imag_sum/1  "xlsub5_fir_tap1_image"
  fir_tap1/1(a_out) -> real_out1/1
  real1/1 -> fir_tap1/1(a)
  imag1/1 -> fir_tap1/2(b)
  fir_tap1/2(b_out) -> imag_out1/1
  fir_tap1/3(real) -> real_sum/1  "xlsub5_fir_tap1_real"

== system xblock_half_band_Model/Subsystem/parallel_fir3/f0pf1/fir_col2 ==
  real1 : Inport
  imag1 : Inport  Port=2
  fir_tap1 : Subsystem
  real_out1 : Outport
  imag_out1 : Outport  Port=2
  real_sum : Outport  Port=3
  imag_sum : Outport  Port=4
  wires:
  fir_tap1/4(imag) -> imag_sum/1  "xlsub5_fir_tap1_image"
  fir_tap1/1(a_out) -> real_out1/1
  real1/1 -> fir_tap1/1(a)
  imag1/1 -> fir_tap1/2(b)
  fir_tap1/2(b_out) -> imag_out1/1
  fir_tap1/3(real) -> real_sum/1  "xlsub5_fir_tap1_real"

== system xblock_half_band_Model/Subsystem/parallel_fir3/f0pf1/fir_col3 ==
  real1 : Inport
  imag1 : Inport  Port=2
  fir_tap1 : Subsystem
  real_out1 : Outport
  imag_out1 : Outport  Port=2
  real_sum : Outport  Port=3
  imag_sum : Outport  Port=4
  wires:
  fir_tap1/4(imag) -> imag_sum/1  "xlsub5_fir_tap1_image"
  fir_tap1/1(a_out) -> real_out1/1
  real1/1 -> fir_tap1/1(a)
  imag1/1 -> fir_tap1/2(b)
  fir_tap1/2(b_out) -> imag_out1/1
  fir_tap1/3(real) -> real_sum/1  "xlsub5_fir_tap1_real"

== system xblock_half_band_Model/Subsystem/parallel_fir3/f0pf1/fir_col4 ==
  real1 : Inport
  imag1 : Inport  Port=2
  fir_tap1 : Subsystem
  real_out1 : Outport
  imag_out1 : Outport  Port=2
  real_sum : Outport  Port=3
  imag_sum : Outport  Port=4
  wires:
  fir_tap1/4(imag) -> imag_sum/1  "xlsub5_fir_tap1_image"
  fir_tap1/1(a_out) -> real_out1/1
  real1/1 -> fir_tap1/1(a)
  imag1/1 -> fir_tap1/2(b)
  fir_tap1/2(b_out) -> imag_out1/1
  fir_tap1/3(real) -> real_sum/1  "xlsub5_fir_tap1_real"

== system xblock_half_band_Model/Subsystem/parallel_fir3/f0pf1/fir_col5 ==
  real1 : Inport
  imag1 : Inport  Port=2
  fir_tap1 : Subsystem
  real_out1 : Outport
  imag_out1 : Outport  Port=2
  real_sum : Outport  Port=3
  imag_sum : Outport  Port=4
  wires:
  fir_tap1/4(imag) -> imag_sum/1  "xlsub5_fir_tap1_image"
  fir_tap1/1(a_out) -> real_out1/1
  real1/1 -> fir_tap1/1(a)
  imag1/1 -> fir_tap1/2(b)
  fir_tap1/2(b_out) -> imag_out1/1
  fir_tap1/3(real) -> real_sum/1  "xlsub5_fir_tap1_real"

== system xblock_half_band_Model/Subsystem/parallel_fir3/f0pf1/imag_sum ==
  sync : Inport
  din_1 : Inport  Port=2
  din_2 : Inport  Port=3
  din_3 : Inport  Port=4
  din_4 : Inport  Port=5
  din_5 : Inport  Port=6
  din_6 : Inport  Port=7
  sync_delay : xbsIndex_r4/Delay  en=off  latency=3  dbl_ovrd=off  reg_retiming=off  block_type=delay
      settings: block_version=11.4
  zero_in : xbsIndex_r4/Constant  arith_type=Unsigned  const=0  n_bits=18  bin_pt=17  explicit_period=off  period=1  equ=P=C  opselect=C  inp2=PCIN>>17  opr=+  inp1=P  carry=CIN  dbl_ovrd=off  block_type=constant
      settings: block_version=11.4
  sync_out : Outport
  dout : Outport  Port=2
  wires:
  sync/1 -> sync_delay/1
  sync_delay/1 -> sync_out/1

== system xblock_half_band_Model/Subsystem/parallel_fir3/f0pf1/real_sum ==
  sync : Inport
  din_1 : Inport  Port=2
  din_2 : Inport  Port=3
  din_3 : Inport  Port=4
  din_4 : Inport  Port=5
  din_5 : Inport  Port=6
  din_6 : Inport  Port=7
  sync_delay : xbsIndex_r4/Delay  en=off  latency=3  dbl_ovrd=off  reg_retiming=off  block_type=delay
      settings: block_version=11.4
  zero_in : xbsIndex_r4/Constant  arith_type=Unsigned  const=0  n_bits=18  bin_pt=17  explicit_period=off  period=1  equ=P=C  opselect=C  inp2=PCIN>>17  opr=+  inp1=P  carry=CIN  dbl_ovrd=off  block_type=constant
      settings: block_version=11.4
  sync_out : Outport
  dout : Outport  Port=2
  wires:
  sync/1 -> sync_delay/1
  sync_delay/1 -> sync_out/1

== system xblock_half_band_Model/Subsystem/parallel_fir3/f1/fir_col1 ==
  real1 : Inport
  imag1 : Inport  Port=2
  fir_tap1 : Subsystem
  real_out1 : Outport
  imag_out1 : Outport  Port=2
  real_sum : Outport  Port=3
  imag_sum : Outport  Port=4
  wires:
  fir_tap1/4(imag) -> imag_sum/1  "xlsub5_fir_tap1_image"
  fir_tap1/1(a_out) -> real_out1/1
  real1/1 -> fir_tap1/1(a)
  imag1/1 -> fir_tap1/2(b)
  fir_tap1/2(b_out) -> imag_out1/1
  fir_tap1/3(real) -> real_sum/1  "xlsub5_fir_tap1_real"

== system xblock_half_band_Model/Subsystem/parallel_fir3/f1/fir_col2 ==
  real1 : Inport
  imag1 : Inport  Port=2
  fir_tap1 : Subsystem
  real_out1 : Outport
  imag_out1 : Outport  Port=2
  real_sum : Outport  Port=3
  imag_sum : Outport  Port=4
  wires:
  fir_tap1/4(imag) -> imag_sum/1  "xlsub5_fir_tap1_image"
  fir_tap1/1(a_out) -> real_out1/1
  real1/1 -> fir_tap1/1(a)
  imag1/1 -> fir_tap1/2(b)
  fir_tap1/2(b_out) -> imag_out1/1
  fir_tap1/3(real) -> real_sum/1  "xlsub5_fir_tap1_real"

== system xblock_half_band_Model/Subsystem/parallel_fir3/f1/fir_col3 ==
  real1 : Inport
  imag1 : Inport  Port=2
  fir_tap1 : Subsystem
  real_out1 : Outport
  imag_out1 : Outport  Port=2
  real_sum : Outport  Port=3
  imag_sum : Outport  Port=4
  wires:
  fir_tap1/4(imag) -> imag_sum/1  "xlsub5_fir_tap1_image"
  fir_tap1/1(a_out) -> real_out1/1
  real1/1 -> fir_tap1/1(a)
  imag1/1 -> fir_tap1/2(b)
  fir_tap1/2(b_out) -> imag_out1/1
  fir_tap1/3(real) -> real_sum/1  "xlsub5_fir_tap1_real"

== system xblock_half_band_Model/Subsystem/parallel_fir3/f1/fir_col4 ==
  real1 : Inport
  imag1 : Inport  Port=2
  fir_tap1 : Subsystem
  real_out1 : Outport
  imag_out1 : Outport  Port=2
  real_sum : Outport  Port=3
  imag_sum : Outport  Port=4
  wires:
  fir_tap1/4(imag) -> imag_sum/1  "xlsub5_fir_tap1_image"
  fir_tap1/1(a_out) -> real_out1/1
  real1/1 -> fir_tap1/1(a)
  imag1/1 -> fir_tap1/2(b)
  fir_tap1/2(b_out) -> imag_out1/1
  fir_tap1/3(real) -> real_sum/1  "xlsub5_fir_tap1_real"

== system xblock_half_band_Model/Subsystem/parallel_fir3/f1/fir_col5 ==
  real1 : Inport
  imag1 : Inport  Port=2
  fir_tap1 : Subsystem
  real_out1 : Outport
  imag_out1 : Outport  Port=2
  real_sum : Outport  Port=3
  imag_sum : Outport  Port=4
  wires:
  fir_tap1/4(imag) -> imag_sum/1  "xlsub5_fir_tap1_image"
  fir_tap1/1(a_out) -> real_out1/1
  real1/1 -> fir_tap1/1(a)
  imag1/1 -> fir_tap1/2(b)
  fir_tap1/2(b_out) -> imag_out1/1
  fir_tap1/3(real) -> real_sum/1  "xlsub5_fir_tap1_real"

== system xblock_half_band_Model/Subsystem/parallel_fir3/f1/fir_col6 ==
  real1 : Inport
  imag1 : Inport  Port=2
  fir_tap1 : Subsystem
  real_out1 : Outport
  imag_out1 : Outport  Port=2
  real_sum : Outport  Port=3
  imag_sum : Outport  Port=4
  wires:
  fir_tap1/4(imag) -> imag_sum/1  "xlsub5_fir_tap1_image"
  fir_tap1/1(a_out) -> real_out1/1
  real1/1 -> fir_tap1/1(a)
  imag1/1 -> fir_tap1/2(b)
  fir_tap1/2(b_out) -> imag_out1/1
  fir_tap1/3(real) -> real_sum/1  "xlsub5_fir_tap1_real"

== system xblock_half_band_Model/Subsystem/parallel_fir3/f1/fir_col7 ==
  real1 : Inport
  imag1 : Inport  Port=2
  fir_tap1 : Subsystem
  real_out1 : Outport
  imag_out1 : Outport  Port=2
  real_sum : Outport  Port=3
  imag_sum : Outport  Port=4
  wires:
  fir_tap1/4(imag) -> imag_sum/1  "xlsub5_fir_tap1_image"
  fir_tap1/1(a_out) -> real_out1/1
  real1/1 -> fir_tap1/1(a)
  imag1/1 -> fir_tap1/2(b)
  fir_tap1/2(b_out) -> imag_out1/1
  fir_tap1/3(real) -> real_sum/1  "xlsub5_fir_tap1_real"

== system xblock_half_band_Model/Subsystem/parallel_fir3/f1/fir_col8 ==
  real1 : Inport
  imag1 : Inport  Port=2
  fir_tap1 : Subsystem
  real_out1 : Outport
  imag_out1 : Outport  Port=2
  real_sum : Outport  Port=3
  imag_sum : Outport  Port=4
  wires:
  fir_tap1/4(imag) -> imag_sum/1  "xlsub5_fir_tap1_image"
  fir_tap1/1(a_out) -> real_out1/1
  real1/1 -> fir_tap1/1(a)
  imag1/1 -> fir_tap1/2(b)
  fir_tap1/2(b_out) -> imag_out1/1
  fir_tap1/3(real) -> real_sum/1  "xlsub5_fir_tap1_real"

== system xblock_half_band_Model/Subsystem/parallel_fir3/f1/imag_sum ==
  sync : Inport
  din_1 : Inport  Port=2
  din_2 : Inport  Port=3
  din_3 : Inport  Port=4
  din_4 : Inport  Port=5
  din_5 : Inport  Port=6
  din_6 : Inport  Port=7
  din_7 : Inport  Port=8
  din_8 : Inport  Port=9
  din_9 : Inport  Port=10
  sync_delay : xbsIndex_r4/Delay  en=off  latency=4  dbl_ovrd=off  reg_retiming=off  block_type=delay
      settings: block_version=11.4
  zero_in : xbsIndex_r4/Constant  arith_type=Unsigned  const=0  n_bits=18  bin_pt=17  explicit_period=off  period=1  equ=P=C  opselect=C  inp2=PCIN>>17  opr=+  inp1=P  carry=CIN  dbl_ovrd=off  block_type=constant
      settings: block_version=11.4
  sync_out : Outport
  dout : Outport  Port=2
  wires:
  sync/1 -> sync_delay/1
  sync_delay/1 -> sync_out/1

== system xblock_half_band_Model/Subsystem/parallel_fir3/f1/real_sum ==
  sync : Inport
  din_1 : Inport  Port=2
  din_2 : Inport  Port=3
  din_3 : Inport  Port=4
  din_4 : Inport  Port=5
  din_5 : Inport  Port=6
  din_6 : Inport  Port=7
  din_7 : Inport  Port=8
  din_8 : Inport  Port=9
  din_9 : Inport  Port=10
  sync_delay : xbsIndex_r4/Delay  en=off  latency=4  dbl_ovrd=off  reg_retiming=off  block_type=delay
      settings: block_version=11.4
  zero_in : xbsIndex_r4/Constant  arith_type=Unsigned  const=0  n_bits=18  bin_pt=17  explicit_period=off  period=1  equ=P=C  opselect=C  inp2=PCIN>>17  opr=+  inp1=P  carry=CIN  dbl_ovrd=off  block_type=constant
      settings: block_version=11.4
  sync_out : Outport
  dout : Outport  Port=2
  wires:
  sync/1 -> sync_delay/1
  sync_delay/1 -> sync_out/1

== system xblock_half_band_Model/Subsystem/parallel_fir/f0/fir_col1/fir_tap1 ==
  a : Inport
  b : Inport  Port=2
  Constant : xbsIndex_r4/Constant  arith_type=Signed (2's comp)  const=1  n_bits=25  bin_pt=24  explicit_period=on  period=1  equ=P=C  opselect=C  inp2=PCIN>>17  opr=+  inp1=P  carry=CIN  dbl_ovrd=off  block_type=constant
      settings: block_version=11.4
  Mult : xbsIndex_r4/Mult  precision=Full  arith_type="Signed  (2's comp)"  n_bits=18  bin_pt=17  quantization=Truncate  overflow=Wrap  en=off  latency=1  dbl_ovrd=off  use_behavioral_HDL=on  opt=Speed  use_embedded=on  optimum_pipeline=off  pipeline=on  use_rpm=off  placement_style=Rectangular shape  block_type=mult
      settings: block_version=11.4
  Mult1 : xbsIndex_r4/Mult  precision=Full  arith_type="Signed  (2's comp)"  n_bits=18  bin_pt=17  quantization=Truncate  overflow=Wrap  en=off  latency=1  dbl_ovrd=off  use_behavioral_HDL=on  opt=Speed  use_embedded=on  optimum_pipeline=off  pipeline=on  use_rpm=off  placement_style=Rectangular shape  block_type=mult
      settings: block_version=11.4
  Register : xbsIndex_r4/Register  init=0  rst=off  en=off  dbl_ovrd=off  block_type=register
      settings: block_version=11.4
  Register1 : xbsIndex_r4/Register  init=0  rst=off  en=off  dbl_ovrd=off  block_type=register
      settings: block_version=11.4
  a_out : Outport
  b_out : Outport  Port=2
  real : Outport  Port=3
  imag : Outport  Port=4
  wires:
  Constant/1 -> Mult/1, Mult1/1
  a/1 -> Mult1/2, Register/1
  b/1 -> Register1/1, Mult/2
  Register/1 -> a_out/1
  Mult/1 -> imag/1
  Mult1/1 -> real/1
  Register1/1 -> b_out/1
